simulink model "hdltest"  (R2021a)
settings: Solver=VariableStepAuto  StartTime=0.0  StopTime=2  RelTol=1e-3
libraries: spspowerguiLib x1
settings Model: Creator=Dell  LastModifiedBy=Dell

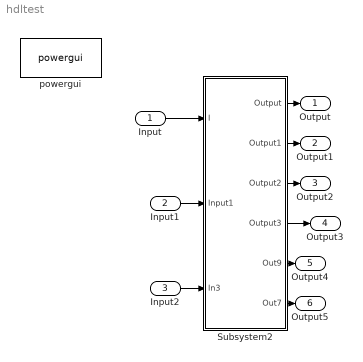
== system hdltest ==
  Input : Inport
  Input1 : Inport  Port=2
  Input2 : Inport  Port=3
  Subsystem2 : Subsystem
  powergui : spspowerguiLib/powergui  Priority=1  SimulationMode=Discrete  SampleTime=5e-6  frequency=60  Iterations=50  frequencyindice=60  Pbase=100e6  ErrMax=1e-4  UnitsV=kV  UnitsW=MW  buscounter=0  FunctionMessages=off  echomessages=off  EnableUseOfTLC=off  CurrentSourceSwitches=off  DisableSnubberDevices=off  DisableRonSwitches=off  DisableVfSwitches=off  DisplayEquations=off  AutomaticDiscreteSolvers=off  SolverType=Tustin/Backward Euler (TBE)  Interpol=off  ExternalGateDelay=off  methode=off  Ts=100  x0status=blocks  SPID=on  SwTol=0  HookPort=off  NonlinearTolerance=1e-4  nMaxIteration=100  ContinueOnMaxIteration=off  RestoreLinks=warning  ResistiveCurrentMeasurement=off  Frange=[0:2:500]  Ylog=off  Xlog=on  ShowGrid=off  save=off  variable=ZData  structure=0  ZoomFFT=off  StartTime=0.0  cycles=1  DisplayStyle=1  fundamental=60  FreqAxis=off  MaxFrequency=1000  frequencyindicesteady=1  RmsSteady=1  display=off
  Output : Outport
  Output1 : Outport  Port=2
  Output2 : Outport  Port=3
  Output3 : Outport  Port=4
  Output4 : Outport  Port=5
  Output5 : Outport  Port=6
  wires:
  Input/1 -> Subsystem2/1(I)
  Input2/1 -> Subsystem2/3(In3)
  Input1/1 -> Subsystem2/2(Input1)
  Subsystem2/6(Out7) -> Output5/1
  Subsystem2/5(Out9) -> Output4/1
  Subsystem2/4(Output3) -> Output3/1
  Subsystem2/3(Output2) -> Output2/1
  Subsystem2/2(Output1) -> Output1/1
  Subsystem2/1(Output) -> Output/1

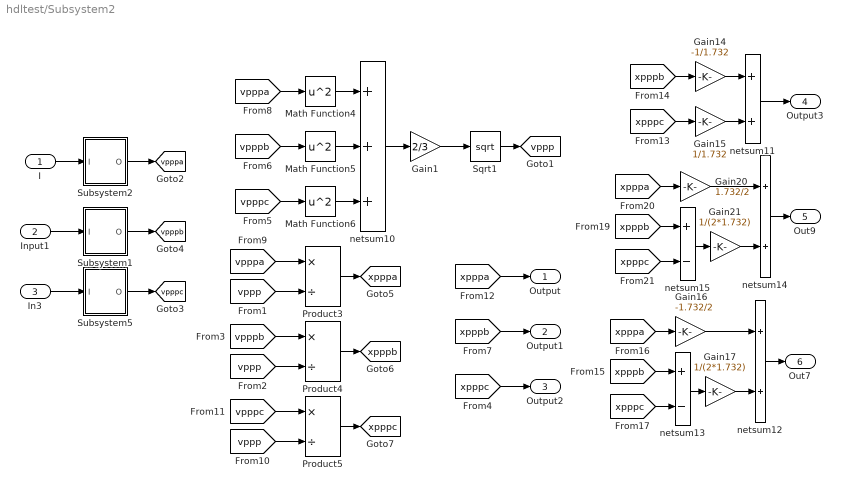
== system hdltest/Subsystem2 ==
  I : Inport
  Input1 : Inport  Port=2
  In3 : Inport  Port=3
  Gain1 : Gain  Gain=2/3
  Gain14 : Gain  Gain=-1/1.732
  Gain15 : Gain  Gain=1/1.732
  Gain16 : Gain  Gain=-1.732/2
  Gain17 : Gain  Gain=1/(2*1.732)
  Gain20 : Gain  Gain=1.732/2
  Gain21 : Gain  Gain=1/(2*1.732)
  Math Function4 : Math  Operator=square  SignedPower=on  SaturateOnIntegerOverflow=on
  Math Function5 : Math  Operator=square  SignedPower=on  SaturateOnIntegerOverflow=on
  Math Function6 : Math  Operator=square  SignedPower=on  SaturateOnIntegerOverflow=on
  Product3 : Product  Inputs=*/  RndMeth=Zero  SaturateOnIntegerOverflow=on
  Product4 : Product  Inputs=*/  RndMeth=Zero  SaturateOnIntegerOverflow=on
  Product5 : Product  Inputs=*/  RndMeth=Zero  SaturateOnIntegerOverflow=on
  Sqrt1 : Sqrt  SaturateOnIntegerOverflow=on
  Subsystem1 : Subsystem
  Subsystem2 : Subsystem
  Subsystem5 : Subsystem
  netsum10 : Sum  Inputs=+++  InputSameDT=on  SaturateOnIntegerOverflow=on  OutDataTypeStr=Inherit: Same as first input
  netsum11 : Sum  InputSameDT=on  SaturateOnIntegerOverflow=on  OutDataTypeStr=Inherit: Same as first input
  netsum12 : Sum  InputSameDT=on  SaturateOnIntegerOverflow=on  OutDataTypeStr=Inherit: Same as first input
  netsum13 : Sum  Inputs=+-  InputSameDT=on  SaturateOnIntegerOverflow=on  OutDataTypeStr=Inherit: Same as first input
  netsum14 : Sum  InputSameDT=on  SaturateOnIntegerOverflow=on  OutDataTypeStr=Inherit: Same as first input
  netsum15 : Sum  Inputs=+-  InputSameDT=on  SaturateOnIntegerOverflow=on  OutDataTypeStr=Inherit: Same as first input
  Output : Outport
  Output1 : Outport  Port=2
  Output2 : Outport  Port=3
  Output3 : Outport  Port=4
  Out9 : Outport  Port=5
  Out7 : Outport  Port=6
  tag scope: vppp=global, vpppa=global, vpppb=global, vpppc=global, xpppa=global, xpppb=global, xpppc=global
  wires:
  Math Function4/1 -> netsum10/1
  Math Function5/1 -> netsum10/2
  Math Function6/1 -> netsum10/3
  netsum10/1 -> Gain1/1
  Sqrt1/1 -> [vppp]
  I/1 -> Subsystem2/1(I)
  In3/1 -> Subsystem5/1(I)
  Input1/1 -> Subsystem1/1(I)
  [vpppb] -> Math Function5/1
  [vpppa] -> Math Function4/1
  [vpppc] -> Math Function6/1
  [vpppa] -> Product3/1
  [vppp] -> Product3/2
  [vppp] -> Product4/2
  [vpppb] -> Product4/1
  [vpppc] -> Product5/1
  [vppp] -> Product5/2
  Product3/1 -> [xpppa]
  Product4/1 -> [xpppb]
  Product5/1 -> [xpppc]
  [xpppa] -> Output/1
  [xpppb] -> Output1/1
  [xpppc] -> Output2/1
  [xpppb] -> Gain14/1
  Gain14/1 -> netsum11/1
  Gain15/1 -> netsum11/2
  [xpppc] -> Gain15/1
  netsum11/1 -> Output3/1
  netsum14/1 -> Out9/1
  [xpppb] -> netsum15/1
  Gain21/1 -> netsum14/2
  Gain20/1 -> netsum14/1
  [xpppa] -> Gain20/1
  [xpppc] -> netsum15/2
  netsum15/1 -> Gain21/1
  netsum13/1 -> Gain17/1
  [xpppc] -> netsum13/2
  [xpppa] -> Gain16/1
  Gain16/1 -> netsum12/1
  Gain17/1 -> netsum12/2
  [xpppb] -> netsum13/1
  netsum12/1 -> Out7/1
  Gain1/1 -> Sqrt1/1
  Subsystem2/1(O) -> [vpppa]
  Subsystem1/1(O) -> [vpppb]
  Subsystem5/1(O) -> [vpppc]

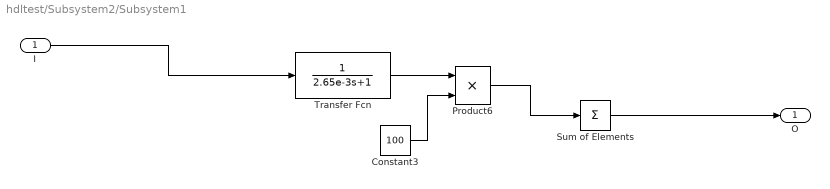
== system hdltest/Subsystem2/Subsystem1 ==
  I : Inport
  Constant3 : Constant  Value=100
  Product6 : Product  RndMeth=Zero
  Sum of Elements : Sum  Inputs=+
  Transfer Fcn : TransferFcn  Denominator=[2.65e-3 1]
  O : Outport
  wires:
  Product6/1 -> Sum of Elements/1
  Constant3/1 -> Product6/2
  Transfer Fcn/1 -> Product6/1
  I/1 -> Transfer Fcn/1
  Sum of Elements/1 -> O/1

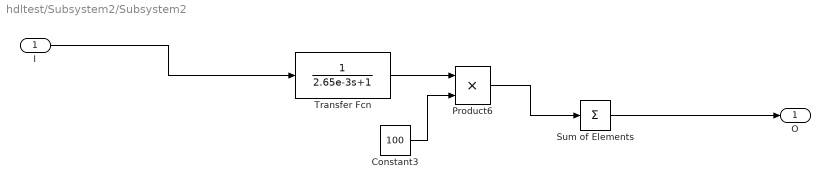
== system hdltest/Subsystem2/Subsystem2 ==
  I : Inport
  Constant3 : Constant  Value=100
  Product6 : Product  RndMeth=Zero
  Sum of Elements : Sum  Inputs=+
  Transfer Fcn : TransferFcn  Denominator=[2.65e-3 1]
  O : Outport
  wires:
  Product6/1 -> Sum of Elements/1
  Constant3/1 -> Product6/2
  Transfer Fcn/1 -> Product6/1
  I/1 -> Transfer Fcn/1
  Sum of Elements/1 -> O/1

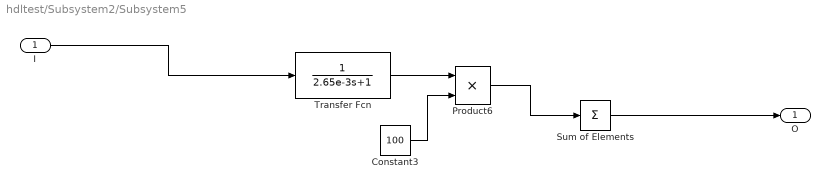
== system hdltest/Subsystem2/Subsystem5 ==
  I : Inport
  Constant3 : Constant  Value=100
  Product6 : Product  RndMeth=Zero
  Sum of Elements : Sum  Inputs=+
  Transfer Fcn : TransferFcn  Denominator=[2.65e-3 1]
  O : Outport
  wires:
  Sum of Elements/1 -> O/1
  I/1 -> Transfer Fcn/1
  Transfer Fcn/1 -> Product6/1
  Constant3/1 -> Product6/2
  Product6/1 -> Sum of Elements/1
